simulink model "STOICAL_example_3_Step02_ActivateSTOICAL"  (R2014b)
settings: Solver=ode4  StartTime=0.0  StopTime=1  FixedStep=50E-6  RelTol=1e-3
model workspace (MAT data in the model file):
  STOVICAL.SignalSaveOptions.ReturnWorkspaceOutputs = 'on'
  STOVICAL.SignalSaveOptions.ReturnWorkspaceOutputsName = 'simout_obj'
  STOVICAL.SignalSaveOptions.SignalLogging = 'on'
  STOVICAL.SignalSaveOptions.SignalLoggingSaveFormat = 'Dataset'
  STOVICAL.SignalSaveOptions.SignalLoggingName = 'STOVICAL_LoggedSignals'
  STOVICAL.ParameterDefinition.BlkNameFull{1} = 'Proportional Element
    | #PARAM#P'
  STOVICAL.ParameterDefinition.BlkNameFull{2} = 'Integral Element
    | #PARAM#I'
  STOVICAL.ParameterDefinition.BlkNameFull{3} = 'Proportional Element
    | #PARAM#P'
  STOVICAL.ParameterDefinition.BlkNameFull{4} = 'Step amplitude
    | #PARAM#Amplitude'
  STOVICAL.ParameterDefinition.BlkNameFull{5} = 'Dynamic System
    | #PARAM#w0#damp'
  STOVICAL.ParameterDefinition.BlkNameFull{6} = 'Static System
    | modelled
    | by gain block
    | #PARAM#SystemGain'
  STOVICAL.ParameterDefinition.BlkNameFull{7} = 'Dynamic System
    | #PARAM#w0#damp'
  STOVICAL.ParameterDefinition.BlkNameShort{1} = 'Proportional Element
    | '
  STOVICAL.ParameterDefinition.BlkNameShort{2} = 'Integral Element
    | '
  STOVICAL.ParameterDefinition.BlkNameShort{3} = 'Proportional Element
    | '
  STOVICAL.ParameterDefinition.BlkNameShort{4} = 'Step amplitude
    | '
  STOVICAL.ParameterDefinition.BlkNameShort{5} = 'Dynamic System
    | '
  STOVICAL.ParameterDefinition.BlkNameShort{6} = 'Static System
    | modelled
    | by gain block
    | '
  STOVICAL.ParameterDefinition.BlkNameShort{7} = 'Dynamic System
    | '
  STOVICAL.ParameterDefinition.BlkHandle = [9.00207519531; 15.0020751953; 17.0020751953; 1948.00512695; 1955.00500488; 1961.00366211; 1955.00500488]
  STOVICAL.ParameterDefinition.ParamName = {'P'; 'I'; 'P'; 'Amplitude'; 'w0'; 'SystemGain'; 'damp'}
  STOVICAL.ParameterDefinition.BlkPath{1} = 'STOICAL_example_3_Step02_ActivateSTOICAL/#UNIT#Controller/P-controller
    | #DEF#/Proportional Element
    | #PARAM#P'
  STOVICAL.ParameterDefinition.BlkPath{2} = 'STOICAL_example_3_Step02_ActivateSTOICAL/#UNIT#Controller/PI-controller/Integral Element
    | #PARAM#I'
  STOVICAL.ParameterDefinition.BlkPath{3} = 'STOICAL_example_3_Step02_ActivateSTOICAL/#UNIT#Controller/PI-controller/Proportional Element
    | #PARAM#P'
  STOVICAL.ParameterDefinition.BlkPath{4} = 'STOICAL_example_3_Step02_ActivateSTOICAL/#UNIT#Stimulus/Step amplitude
    | #PARAM#Amplitude'
  STOVICAL.ParameterDefinition.BlkPath{5} = 'STOICAL_example_3_Step02_ActivateSTOICAL/#UNIT#System/Dynamic System
    | #PARAM#w0#damp'
  STOVICAL.ParameterDefinition.BlkPath{6} = 'STOICAL_example_3_Step02_ActivateSTOICAL/#UNIT#System/Static System
    | modelled
    | by gain block
    | #PARAM#SystemGain'
  STOVICAL.ParameterDefinition.BlkPath{7} = 'STOICAL_example_3_Step02_ActivateSTOICAL/#UNIT#System/Dynamic System
    | #PARAM#w0#damp'
  STOVICAL.ParameterDefinition.BlkType = {'Gain'; 'Gain'; 'Gain'; 'Constant'; 'SubSystem'; 'Gain'; 'SubSystem'}
  STOVICAL.ParameterDefinition.BlkMaskType = {''; ''; ''; ''; ''; ''; ''}
  STOVICAL.ParameterDefinition.ParentalBlockPath{1} = 'STOICAL_example_3_Step02_ActivateSTOICAL/#UNIT#Controller/P-controller
    | #DEF#'
  STOVICAL.ParameterDefinition.ParentalBlockPath{2} = 'STOICAL_example_3_Step02_ActivateSTOICAL/#UNIT#Controller/PI-controller'
  STOVICAL.ParameterDefinition.ParentalBlockPath{3} = 'STOICAL_example_3_Step02_ActivateSTOICAL/#UNIT#Controller/PI-controller'
  STOVICAL.ParameterDefinition.ParentalBlockPath{4} = 'STOICAL_example_3_Step02_ActivateSTOICAL/#UNIT#Stimulus'
  STOVICAL.ParameterDefinition.ParentalBlockPath{5} = 'STOICAL_example_3_Step02_ActivateSTOICAL/#UNIT#System'
  STOVICAL.ParameterDefinition.ParentalBlockPath{6} = 'STOICAL_example_3_Step02_ActivateSTOICAL/#UNIT#System'
  STOVICAL.ParameterDefinition.ParentalBlockPath{7} = 'STOICAL_example_3_Step02_ActivateSTOICAL/#UNIT#System'
  STOVICAL.ParameterDefinition.ParentalBlockHandle = [7.00207519531; 13.0062255859; 13.0062255859; 1945.00366211; 1953.00268555; 1953.00268555; 1953.00268555]
  STOVICAL.ParameterDefinition.Belongs2SubsystemHdl = [7.00207519531; 13.0062255859; 13.0062255859; 1945.00366211; 1955.00500488; 1953.00268555; 1955.00500488]
  STOVICAL.ParameterDefinition.NrParams = 7
  STOVICAL.ParameterDefinition.BlkField2Set = {'Gain'; 'Gain'; 'Gain'; 'Value'; 'w0'; 'Gain'; 'damp'}
  STOVICAL.ParameterDefinition.BlkFieldSyntax = {'#'; '#'; '#'; '#'; '#'; '#'; '#'}
  STOVICAL.ParameterDefinition.ParamVariable = {'param_3c9c89c931886ed3127a48daf9f95107'; 'param_a6ec8c1abcd3e361be1ac1b9cb9444f5'; 'param_5f7e5cb4a090d61c0e7cb0acc03122bf'; 'param_198a5ba83d87bd2227ff7bec4eafe564'; 'param_cc726f90f8a3943432e26d7ec8664179'; 'param_5d6f2ad7a9e66dc7adc2c2fe631bc1c7'; 'param_b7b38d61b0a2fdc551dbbf041a783640'}
  STOVICAL.ParameterDefinition.LabelPath = {'#Controller#P'; '#Controller#I'; '#Controller#P'; '#Stimulus#Amplitude'; '#System#w0'; '#System#SystemGain'; '#System#damp'}
  STOVICAL.ParameterDefinition.ParamDefaultValue = {'10'; '1/100'; '10'; '2'; '50'; '5'; '1/sqrt(2)'}
  STOVICAL.SignalDefinition.ParentalBlockPath = {'STOICAL_example_3_Step02_ActivateSTOICAL'; 'STOICAL_example_3_Step02_ActivateSTOICAL'; 'STOICAL_example_3_Step02_ActivateSTOICAL'}
  STOVICAL.SignalDefinition.ParentalBlockHandle = [3.00317382812; 3.00317382812; 3.00317382812]
  STOVICAL.SignalDefinition.NameInDiagram = {'#SIG#u'; '#SIG#stimulus'; '#SIG#response'}
  STOVICAL.SignalDefinition.SourceBlockPath = {'STOICAL_example_3_Step02_ActivateSTOICAL/#UNIT#Controller'; 'STOICAL_example_3_Step02_ActivateSTOICAL/#UNIT#Stimulus'; 'STOICAL_example_3_Step02_ActivateSTOICAL/#UNIT#System'}
  STOVICAL.SignalDefinition.SourceBlockPort = [1; 1; 1]
  STOVICAL.SignalDefinition.SourceBlockHandle = [5.04992675781; 1945.00366211; 1953.00268555]
  STOVICAL.SignalDefinition.Handle = [1980.00158691; 1974.00354004; 1977.00109863]
  STOVICAL.SignalDefinition.NrSig = 3
  STOVICAL.SignalDefinition.NameOfLogVar = {'logsig_5127ef3fcd5d85aa8d97810318f74f95'; 'logsig_17c77b4b67075e6c5b34308ff6d10315'; 'logsig_cd8f6ce6d7b25f261afaaa2903816a10'}
  STOVICAL.SignalDefinition.NameOfLogVarMode = {'SignalName'; 'Custom'; 'Custom'}
  STOVICAL.SignalDefinition.DoLog = [0; 1; 1]
  STOVICAL.SignalDefinition.LabelPath = {'#u'; '#stimulus'; '#response'}
  STOVICAL.VariantDefinition.NodeHandle = [3.00317382812; 5.04992675781; 1945.00366211; 1953.00268555; 7.00207519531; 13.0062255859; 1955.00500488]
  STOVICAL.VariantDefinition.NodeName{1} = 'STOICAL_example_3_Step02_ActivateSTOICAL'
  STOVICAL.VariantDefinition.NodeName{2} = '#UNIT#Controller'
  STOVICAL.VariantDefinition.NodeName{3} = '#UNIT#Stimulus'
  STOVICAL.VariantDefinition.NodeName{4} = '#UNIT#System'
  STOVICAL.VariantDefinition.NodeName{5} = 'P-controller
    | #DEF#'
  STOVICAL.VariantDefinition.NodeName{6} = 'PI-controller'
  STOVICAL.VariantDefinition.NodeName{7} = 'Dynamic System
    | #PARAM#w0#damp'
  STOVICAL.VariantDefinition.IsVariantSubsystem = [0; 1; 0; 0; 0; 0; 0]
  STOVICAL.VariantDefinition.NodeLevel = [1; 2; 2; 2; 3; 3; 3]
  STOVICAL.VariantDefinition.NodePath{1} = 'STOICAL_example_3_Step02_ActivateSTOICAL'
  STOVICAL.VariantDefinition.NodePath{2} = 'STOICAL_example_3_Step02_ActivateSTOICAL/#UNIT#Controller'
  STOVICAL.VariantDefinition.NodePath{3} = 'STOICAL_example_3_Step02_ActivateSTOICAL/#UNIT#Stimulus'
  STOVICAL.VariantDefinition.NodePath{4} = 'STOICAL_example_3_Step02_ActivateSTOICAL/#UNIT#System'
  STOVICAL.VariantDefinition.NodePath{5} = 'STOICAL_example_3_Step02_ActivateSTOICAL/#UNIT#Controller/P-controller
    | #DEF#'
  STOVICAL.VariantDefinition.NodePath{6} = 'STOICAL_example_3_Step02_ActivateSTOICAL/#UNIT#Controller/PI-controller'
  STOVICAL.VariantDefinition.NodePath{7} = 'STOICAL_example_3_Step02_ActivateSTOICAL/#UNIT#System/Dynamic System
    | #PARAM#w0#damp'
  STOVICAL.VariantDefinition.IsVariant = [0; 0; 0; 0; 1; 1; 0]
  STOVICAL.VariantDefinition.VSNodeIdxofVariant = [0; 0; 0; 0; 2; 2; 0]
  STOVICAL.VariantDefinition.VSVariantsCount = [0; 2; 0; 0; 0; 0; 0]
  STOVICAL.VariantDefinition.VSVariantsBlkHdls = {[]; [7.00207519531; 13.0062255859]; []; []; []; []; []}
  STOVICAL.VariantDefinition.VSVariantsNodeIdx = {[]; [5; 6]; []; []; []; []; []}
  STOVICAL.VariantDefinition.VSControlVariable = {[]; 'varsys_cond_9012b32a464bd3373daa07b1fc176436'; []; []; []; []; []}
  STOVICAL.VariantDefinition.VSVariantHasNr = [0; 0; 0; 0; 1; 2; 0]
  STOVICAL.VariantDefinition.IsDefaultVariant = [0; 0; 0; 0; 1; 0; 0]
  STOVICAL.VariantDefinition.VSDefaultVariantNr = [0; 1; 0; 0; 0; 0; 0]
  STOVICAL.VariantDefinition.LabelPath = {[]; '#Controller'; []; []; []; []; []}
  param_ec6e274da2c23e664dfdc874ac252818 = '2'
  param_afc1e04cc1c158b687408e5b6ea19d06 = '5'
  param_9ba35cf139ae8d049712606822772694 = '2'
  param_518f5dd230dc6df197dc8805b8657145 = '50'
  param_b7a2875e19f2aaba8a6b37e383b6fdf1 = '5'
  param_13ac9ebe924e8dfd32ee0d3deb3cd2af = '1/sqrt(2)'
undefined symbols (not defined in the file): param_198a5ba83d87bd2227ff7bec4eafe564, param_3c9c89c931886ed3127a48daf9f95107, param_5d6f2ad7a9e66dc7adc2c2fe631bc1c7, param_5f7e5cb4a090d61c0e7cb0acc03122bf, param_a6ec8c1abcd3e361be1ac1b9cb9444f5, param_b7b38d61b0a2fdc551dbbf041a783640, param_cc726f90f8a3943432e26d7ec8664179
settings Model: Creator=Wippenbeck  LastModifiedBy=Wippenbeck
settings DataIOCC: ReturnWorkspaceOutputs=on  SignalLoggingName=STOVICAL_LoggedSignals  ReturnWorkspaceOutputsName=simout_obj

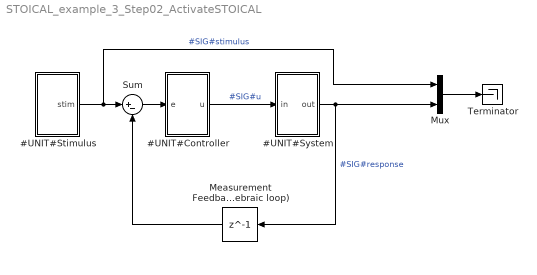
== system STOICAL_example_3_Step02_ActivateSTOICAL ==
  #UNIT#Controller : Subsystem  Variant=on
  #UNIT#Stimulus : Subsystem
  #UNIT#System : Subsystem
  Measurement Feedback (avoids algebraic loop) : Delay  DelayLength=1  InitialCondition=0
  Mux : Mux  Inputs=2
  Sum : Sum  Inputs=|+-
  Terminator : Terminator
  wires:
  Mux/1 -> Terminator/1
  #UNIT#Stimulus/1(stim) -> Sum/1, Mux/1  "#SIG#stimulus"
  #UNIT#System/1(out) -> Measurement Feedback (avoids algebraic loop)/1, Mux/2  "#SIG#response"
  Measurement Feedback (avoids algebraic loop)/1 -> Sum/2
  Sum/1 -> #UNIT#Controller/1(e)
  #UNIT#Controller/1(u) -> #UNIT#System/1(in)  "#SIG#u"

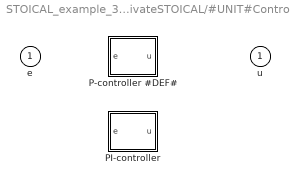
== system STOICAL_example_3_Step02_ActivateSTOICAL/#UNIT#Controller ==
  e : Inport
  P-controller #DEF# : Subsystem  VariantControl=varsys_cond_9012b32a464bd3373daa07b1fc176436 == 1
  PI-controller : Subsystem  VariantControl=varsys_cond_9012b32a464bd3373daa07b1fc176436 == 2
  u : Outport

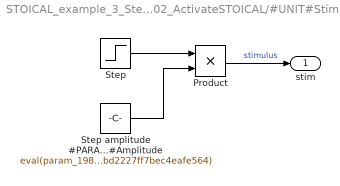
== system STOICAL_example_3_Step02_ActivateSTOICAL/#UNIT#Stimulus ==
  Product : Product
  Step : Step  Time=0.1  SampleTime=0
  Step amplitude #PARAM#Amplitude : Constant  Value=eval(param_198a5ba83d87bd2227ff7bec4eafe564)
  stim : Outport
  wires:
  Step amplitude #PARAM#Amplitude/1 -> Product/2
  Product/1 -> stim/1  "stimulus"
  Step/1 -> Product/1

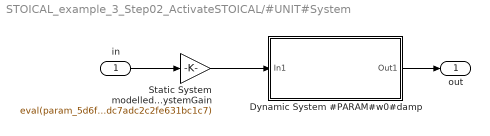
== system STOICAL_example_3_Step02_ActivateSTOICAL/#UNIT#System ==
  in : Inport
  Dynamic System #PARAM#w0#damp : Subsystem  mask{w0=eval(param_cc726f90f8a3943432e26d7ec8664179), damp=eval(param_b7b38d61b0a2fdc551dbbf041a783640)}
      mask prompts: w0 "Natural frequency w0 [rad/s]"; damp "Damping zeta [1]"
      mask help:
      | Dynamical system of the form
      |
      | G(s) = w0^2 / (s^2 + 2*zeta*w0*s + wo^2)
  Static System modelled by gain block #PARAM#SystemGain : Gain  Gain=eval(param_5d6f2ad7a9e66dc7adc2c2fe631bc1c7)
  out : Outport
  wires:
  in/1 -> Static System modelled by gain block #PARAM#SystemGain/1
  Static System modelled by gain block #PARAM#SystemGain/1 -> Dynamic System #PARAM#w0#damp/1(In1)
  Dynamic System #PARAM#w0#damp/1(Out1) -> out/1

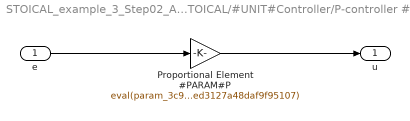
== system STOICAL_example_3_Step02_ActivateSTOICAL/#UNIT#Controller/P-controller #DEF# ==
  e : Inport
  Proportional Element #PARAM#P : Gain  Gain=eval(param_3c9c89c931886ed3127a48daf9f95107)
  u : Outport
  wires:
  Proportional Element #PARAM#P/1 -> u/1
  e/1 -> Proportional Element #PARAM#P/1

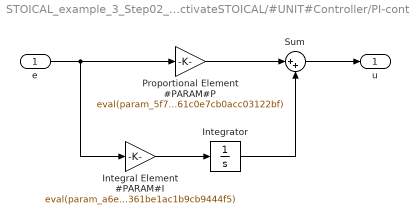
== system STOICAL_example_3_Step02_ActivateSTOICAL/#UNIT#Controller/PI-controller ==
  e : Inport
  Integral Element #PARAM#I : Gain  Gain=eval(param_a6ec8c1abcd3e361be1ac1b9cb9444f5)
  Integrator : Integrator
  Proportional Element #PARAM#P : Gain  Gain=eval(param_5f7e5cb4a090d61c0e7cb0acc03122bf)
  Sum : Sum  Inputs=|++
  u : Outport
  wires:
  Proportional Element #PARAM#P/1 -> Sum/1
  e/1 -> Integral Element #PARAM#I/1, Proportional Element #PARAM#P/1
  Sum/1 -> u/1
  Integrator/1 -> Sum/2
  Integral Element #PARAM#I/1 -> Integrator/1

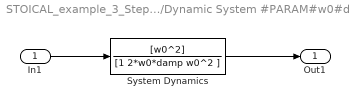
== system STOICAL_example_3_Step02_ActivateSTOICAL/#UNIT#System/Dynamic System #PARAM#w0#damp ==
  In1 : Inport
  System Dynamics : TransferFcn  Numerator=[w0^2]  Denominator=[1 2*w0*damp w0^2 ]
  Out1 : Outport
  wires:
  System Dynamics/1 -> Out1/1
  In1/1 -> System Dynamics/1
